simulink model "ROS_OAC_HOSM_Circular"  (R2018b)
settings: Solver=FixedStepAuto  StartTime=0.0  StopTime=inf  FixedStep=0.02  RelTol=1e-3
model workspace (MAT data in the model file):
  a = Simulink.Parameter
  a.DataType = 'auto'
  a.Dimensions = [0 0]
undefined symbols (not defined in the file): Angular, Linear, magnitude
libraries: simulink x3, robotlib x3
settings Model: Creator=Joru Fua  LastModifiedBy=Joru
settings OptimizationCC: EnhancedBackFolding=on  PassReuseOutputArgsAs=Individual arguments  MaxStackSize=64  OptimizeBlockOrder=speed  DifferentSizesBufferReuse=on  OptimizationCustomize=off
settings DebuggingCC: ParameterTunabilityLossMsg=error
settings HardwareCC: ProdBitPerPointer=32  ProdBitPerSizeT=32  ProdBitPerPtrDiffT=32  ProdLargestAtomicFloat=None  ProdIntDivRoundTo=Undefined  ProdEndianess=Unspecified  ProdWordSize=32  ProdHWDeviceType=Generic->Unspecified (assume 32-bit Generic)
settings SFSimCC: SimUseLocalCustomCode=off  MATLABDynamicMemAlloc=off
settings RTWCC: SystemTargetFile=ert.tlc  HardwareBoard=Robot Operating System (ROS)  TLCOptions="-aInlineSetEventsForThisBaseRateFcn=TLC_FALSE -aSuppressMultiTaskScheduler=TLC_FALSE  -aRateBasedStepFcn=0"  TemplateMakefile=ert_default_tmf  GenerateReport=on  RTWUseLocalCustomCode=off  Toolchain=Catkin  IncludeHyperlinkInReport=on  LaunchReport=on  TargetLang=C++  GenerateTraceInfo=on  GenerateTraceReport=on  GenerateTraceReportSl=on  GenerateTraceReportSf=on  GenerateTraceReportEml=on
settings CodeAppCC: ForceParamTrailComments=on  IgnoreCustomStorageClasses=off  OperatorAnnotations=on  SimulinkDataObjDesc=on  SFDataObjDesc=on  InsertBlockDesc=on
settings ERTTargetCC: SupportContinuousTime=on

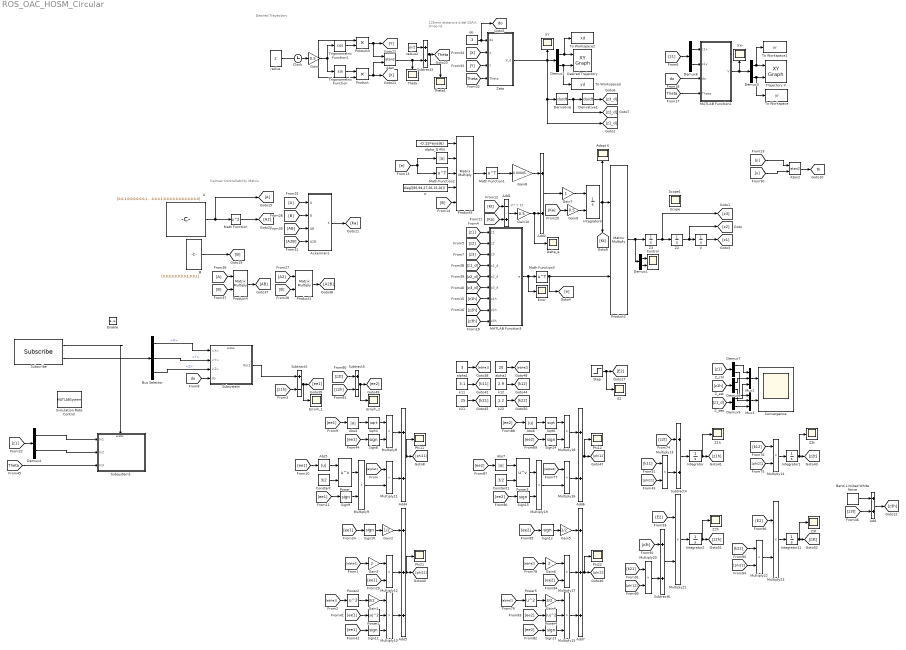
== system ROS_OAC_HOSM_Circular ==
  note: K* = Kt
  note: Kalman Controllability Matrix
  note: Desired Trayectory
  note: 125mm distancia d del SSAV;
      | 0<do<d
  Enable : EnablePort
  A : Constant  Value=[0,0,1,0,0,0;0,0,0,1,0,0;0,0,0,0,1,0;0,0,0,0,0,1;0,0,0,0,0,0;0,0,0,0,0,0]
  Abs{,4..7} (5 alike) : Abs
  Ackerman1 : MATLAB Function  TreatAsAtomicUnit=on
  Adapt K : Scope
  Add{,2,4,6} (4 alike) : Sum
  Add1 : Sum  Inputs=-+
  Add5 : Sum  Inputs=+++
  Add7 : Sum  Inputs=+++
  Atan : Trigonometry  Operator=atan2
  Atan2 : Trigonometry  Operator=atan2
  B : Constant  Value=[0,0;0,0;0,0;0,0;1,0;0,1]  VectorParams1D=off
  Band-Limited White Noise : simulink/Sources/Band-Limited White Noise  Cov=[0.00001]  Ts=0.02  seed=[23341]
  Bus Selector : BusSelector  OutputSignals=Pose.Pose.Position.X,Pose.Pose.Position.Y,Twist.Twist.Angular.Z
  Clock : Clock
  Constant : Constant  Value=3/2
  Constant1 : Constant  Value=3/2
  Control : Scope  NumInputPorts=2
  Convergence : Scope  NumInputPorts=2
  Delta_e : Scope
  Demux{1..4,6..9} (8 alike) : Demux  Outputs=2
  Derivative : Derivative
  Derivative1 : Derivative
  Desired Trajectory : simulink/Sinks/XY Graph  xmin=-5  xmax=5  ymin=-5  ymax=5  st=.1
  E2 : Scope
  Error : Scope
  Errorh_1 : Scope
  Errorh_2 : Scope
  Gain : Gain  Gain=0.5
  Gain1 : Gain  Gain=3/2
  Gain10 : Gain  Gain=0.5
  Gain2 : Gain  Gain=1/2
  Gain3 : Gain  Gain=2
  Gain4 : Gain  Gain=3/2
  Gain5 : Gain  Gain=1/2
  Gain6 : Gain  Gain=2
  Gain7 : Gain
  Gain8 : Gain  Gain=0.00005
  Gain9 : Gain  Gain=0.5
  Integrator{,1..2,11} (4 alike) : Integrator  InitialCondition=[0;0]
  Integrator3 : Integrator  InitialConditionSource=external  InitialCondition=[0.3148,1.3520,2.7441,3.3146,2.4323,0.9017;0.0296,0.1557,0.4075,0.7024,0.9017,1.0442];
  MATLAB Function2 : MATLAB Function  TreatAsAtomicUnit=on
  MATLAB Function3 : MATLAB Function  TreatAsAtomicUnit=on
  Math Function : Math  Operator=square  SaturateOnIntegerOverflow=on
  Math Function1 : Math  Operator=transpose  SaturateOnIntegerOverflow=on
  Math Function2 : Math  Operator=transpose  SaturateOnIntegerOverflow=on
  Math Function3 : Math  Operator=transpose  SaturateOnIntegerOverflow=on
  Multiply10 : Product  Inputs=3
  Multiply{8..9,11..14,16..23} (14 alike) : Product
  Multiply15 : Product  Inputs=3
  Mux2 : Mux  Inputs=3
  Mux3 : Mux  Inputs=3
  P : Constant  Value=diag([85,94,27,26,15,26])
  Phi{11..12,21..22} (4 alike) : Scope
  Power : Math  Operator=pow  SaturateOnIntegerOverflow=on
  Power1 : Math  Operator=magnitude^2  SaturateOnIntegerOverflow=on
  Power2 : Math  Operator=square  SaturateOnIntegerOverflow=on
  Power3 : Math  Operator=pow  SaturateOnIntegerOverflow=on
  Power4 : Math  Operator=magnitude^2  SaturateOnIntegerOverflow=on
  Power5 : Math  Operator=square  SaturateOnIntegerOverflow=on
  Product : Product
  Product1 : Product  Multiplication=Matrix(*)
  Product2 : Product  Multiplication=Matrix(*)
  Product3 : Product
  Product4 : Product  Multiplication=Matrix(*)
  Product5 : Product  Inputs=5  Multiplication=Matrix(*)
  Sign{8..15} (8 alike) : Signum
  Simulation Rate Control : MATLABSystem  System=ExampleHelperSimulationRateControl  SampleTime=0.02
      mask Type: ExampleHelperSimulationRateControl
      mask Display: disp('Rate Control');
  Sqrt4 : Sqrt  SaturateOnIntegerOverflow=on
  Sqrt6 : Sqrt  SaturateOnIntegerOverflow=on
  Step : Step  Time=0.000000001  SampleTime=0.02
  Subscribe : robotlib/Subscribe  topicSource=Specify your own  topic=/odom  messageType=nav_msgs/Odometry  sampleTime=-1  messageQueueLength=1
      settings: SourceProductBaseCode=RO
  Subsystem : Subsystem
  Subsystem1 : Subsystem
  Subtract2 : Sum  Inputs=+-
  Subtract3 : Sum
  Subtract4 : Sum
  Subtract5 : Sum  Inputs=+-
  Subtract6 : Sum
  Theta : Scope
  Theta1 : Scope
  To Workspace : ToWorkspace  VariableName=yr  SampleTime=-1
      settings: Save2DSignal=2-D array (concatenate along first dimension)
  To Workspace1 : ToWorkspace  VariableName=xr  SampleTime=-1
      settings: Save2DSignal=2-D array (concatenate along first dimension)
  To Workspace2 : ToWorkspace  VariableName=xd  SampleTime=-1
      settings: Save2DSignal=2-D array (concatenate along first dimension)
  To Workspace3 : ToWorkspace  VariableName=yd  SampleTime=-1
      settings: Save2DSignal=2-D array (concatenate along first dimension)
  Trajectory V : simulink/Sinks/XY Graph  xmin=-5  xmax=5  ymin=-5  ymax=5  st=.1
  Trigonometric Function : Trigonometry
  Trigonometric Function1 : Trigonometry  Operator=cos
  V : Integrator  InitialCondition=[0;0]
  XY : Scope
  XYr : Scope
  Z1h : Scope
  Z2 : Integrator  InitialCondition=[0;0]
  Z2h : Scope
  Z2t : Scope
  Z3 : Integrator  InitialCondition=[0;0]
  Z3t : Scope
  Zeta : MATLAB Function  TreatAsAtomicUnit=on
  alpha1 : Constant  Value=3
  alpha2 : Constant  Value=20
  alpha_Q : Constant  Value=-0.15*eye(6)
  do : Constant  Value=.3
  k11 : Constant  Value=3.1
  k12 : Constant  Value=2.9
  k21 : Constant  Value=.25
  k22 : Constant  Value=1.2
  radius : Constant  Value=2
  radius2 : Constant  Value=pi/2
  Scope : Scope
  Scope1 : Scope
  tag scope: Theta=global, do=global, th=global
  wires:
  Z3/1 -> [z3], Z2/1
  V/1 -> [z1]
  Derivative1/1 -> [z3_d]
  Derivative/1 -> [z2_d], Derivative1/1
  Product2/1 -> Demux1/1, Z3/1
  Zeta/1(V_d) -> Demux2/1, XY/1, Derivative/1, [z1_d]
  [Theta] -> MATLAB Function2/4(Theta)
  [do] -> MATLAB Function2/3(do)
  Demux6/1 -> MATLAB Function2/1(z1x)
  Demux6/2 -> MATLAB Function2/2(z1y)
  Atan/1 -> Subtract3/2, Theta/1
  radius2/1 -> Subtract3/1
  do/1 -> [do], Zeta/1(do)
  Product/1 -> [X], Atan/2
  Clock/1 -> Gain/1
  [Theta] -> Zeta/4(Theta)
  [X] -> Zeta/2(X)
  [Y] -> Zeta/3(Y)
  Gain/1 -> Trigonometric Function/1, Trigonometric Function1/1
  Trigonometric Function/1 -> Product/1
  radius/1 -> Product/2, Product3/1
  Product3/1 -> Atan/1, [Y]
  Trigonometric Function1/1 -> Product3/2
  [A] -> Ackerman1/1(A)
  B/1 -> [B]
  [AB] -> Ackerman1/3(AB)
  [B] -> Product1/2
  [B] -> Ackerman1/2(B)
  Math Function/1 -> [A2]
  [A2B] -> Ackerman1/4(A2B)
  A/1 -> [A], Math Function/1
  [A2] -> Product1/1
  Product1/1 -> [A2B]
  Product4/1 -> [AB]
  [B] -> Product4/2
  [A] -> Product4/1
  [z3] -> MATLAB Function3/3(z3)
  [z2] -> MATLAB Function3/2(z2)
  [z1] -> MATLAB Function3/1(z1)
  [z1_d] -> MATLAB Function3/4(z1_d)
  [z2_d] -> MATLAB Function3/5(z2_d)
  [z3_d] -> MATLAB Function3/6(z3_d)
  MATLAB Function2/1(V) -> Demux3/1, XYr/1
  Demux3/1 -> To Workspace1/1, Trajectory V/1
  Demux3/2 -> To Workspace/1, Trajectory V/2
  Demux2/1 -> Desired Trajectory/1, To Workspace2/1
  Demux2/2 -> To Workspace3/1, Desired Trajectory/2
  Abs4/1 -> Sqrt4/1
  Constant/1 -> Power/2
  Sqrt4/1 -> Multiply8/1
  Sign8/1 -> Multiply8/2
  Power/1 -> Multiply9/1
  Sign9/1 -> Multiply9/2
  Multiply8/1 -> Add4/1
  Add4/1 -> Phi11/1, [phi11]
  Sign10/1 -> Gain2/1
  Gain2/1 -> Add5/1
  Multiply10/1 -> Add5/3
  Sign11/1 -> Multiply10/3
  alpha1/1 -> [alpha1]
  Multiply9/1 -> Multiply11/2
  [alpha1] -> Multiply11/1
  Multiply11/1 -> Add4/2
  [alpha1] -> Gain3/1
  Gain3/1 -> Multiply12/1
  Multiply12/1 -> Add5/2
  Gain1/1 -> Multiply10/1
  Power2/1 -> Gain1/1
  [alpha1] -> Power2/1
  Power1/1 -> Multiply10/2
  Subtract2/1 -> Errorh_1/1, [ee1]
  [ee1] -> Abs4/1
  [ee1] -> Abs5/1
  [ee1] -> Sign9/1
  [ee1] -> Sign10/1
  [ee1] -> Multiply12/2
  [ee1] -> Power1/1
  [ee1] -> Sign11/1
  [ee1] -> Sign8/1
  k11/1 -> [k11]
  Subtract4/1 -> Integrator/1
  Integrator/1 -> Z1h/1, [z1h]
  Multiply14/1 -> Integrator1/1
  Integrator1/1 -> Z2t/1, [z2t]
  k12/1 -> [k12]
  k21/1 -> [k21]
  [ee2] -> Sign14/1
  Add7/1 -> Phi22/1, [phi22]
  [ee2] -> Sign13/1
  [ee2] -> Power4/1
  [ee2] -> Multiply17/2
  [ee2] -> Sign12/1
  [ee2] -> Sign15/1
  [ee2] -> Abs7/1
  [ee2] -> Abs6/1
  Power4/1 -> Multiply15/2
  [alpha2] -> Power5/1
  Power5/1 -> Gain4/1
  Gain4/1 -> Multiply15/1
  Multiply17/1 -> Add7/2
  Gain6/1 -> Multiply17/1
  [alpha2] -> Gain6/1
  Multiply16/1 -> Add6/2
  [alpha2] -> Multiply16/1
  Multiply19/1 -> Multiply16/2
  Sign13/1 -> Multiply15/3
  Multiply15/1 -> Add7/3
  Gain5/1 -> Add7/1
  Sign12/1 -> Gain5/1
  Add6/1 -> Phi12/1, [phi12]
  Multiply18/1 -> Add6/1
  Sign15/1 -> Multiply19/2
  Power3/1 -> Multiply19/1
  Sign14/1 -> Multiply18/2
  Sqrt6/1 -> Multiply18/1
  Constant1/1 -> Power3/2
  Abs6/1 -> Sqrt6/1
  alpha2/1 -> [alpha2]
  Subtract5/1 -> Errorh_2/1, [ee2]
  k22/1 -> [k22]
  [phi11] -> Multiply13/2
  [k11] -> Multiply13/1
  Multiply13/1 -> Subtract4/2
  [z2t] -> Subtract4/1
  [k12] -> Multiply14/1
  [phi21] -> Multiply14/2
  [z3t] -> Subtract6/1
  Multiply20/1 -> Subtract6/2
  [k21] -> Multiply20/1
  [phi12] -> Multiply20/2
  Integrator2/1 -> Z2h/1, [z2h]
  Subtract6/1 -> Multiply21/2
  [E2] -> Multiply21/1
  Multiply21/1 -> Integrator2/1
  [phi22] -> Multiply22/2
  [k22] -> Multiply22/1
  Multiply22/1 -> Multiply23/2
  [E2] -> Multiply23/1
  Integrator11/1 -> [z3t], Z3t/1
  Multiply23/1 -> Integrator11/1
  [z1h] -> MATLAB Function3/7(z1h)
  [z2h] -> MATLAB Function3/8(z2h)
  [z3h] -> MATLAB Function3/9(z3h)
  Step/1 -> E2/1, [E2]
  Add5/1 -> Phi21/1, [phi21]
  [z1h] -> Subtract2/2
  [z2t] -> Subtract5/1
  [z2h] -> Subtract5/2
  Abs5/1 -> Power/1
  Abs7/1 -> Power3/1
  Z2/1 -> [z2], V/1
  Band-Limited White Noise/1 -> Add/1
  Add/1 -> [z3h]
  [z3t] -> Add/2
  Mux2/1 -> Convergence/1
  Mux3/1 -> Convergence/2
  [z1] -> Demux7/1
  [z1h] -> Demux8/1
  [z1_d] -> Demux9/1
  Demux7/1 -> Mux2/1
  Demux8/1 -> Mux2/2
  Demux9/1 -> Mux2/3
  Demux7/2 -> Mux3/1
  Demux9/2 -> Mux3/3
  Demux8/2 -> Mux3/2
  Demux1/1 -> Control/1
  Demux1/2 -> Control/2
  [z1] -> Demux6/1
  Add2/1 -> Gain7/1
  alpha_Q/1 -> Product5/1
  P/1 -> Product5/4
  Integrator3/1 -> Product2/1, Adapt K/1, [Kt]
  [B] -> Product5/5
  Add1/1 -> Gain10/1
  MATLAB Function3/1(e) -> Error/1, Math Function3/1
  Ackerman1/1(K) -> [Ka]
  Product5/1 -> Math Function1/1
  Math Function3/1 -> Product2/2, [e]
  Math Function2/1 -> Product5/3
  [Kt] -> Add1/1
  Math Function1/1 -> Gain8/1
  [Ka] -> Gain9/1
  Gain7/1 -> Integrator3/1
  [Ka] -> Add1/2
  Gain9/1 -> Integrator3/2
  Gain8/1 -> Add2/1
  Gain10/1 -> Delta_e/1, Add2/2
  [e] -> Abs/1, Math Function2/1
  Abs/1 -> Product5/2
  [y] -> Atan2/1
  [x] -> Atan2/2
  Atan2/1 -> [th]
  Subtract3/1 -> Theta1/1, [Theta]
  [z1] -> Demux4/1
  Subscribe/1 -> Subsystem1/Enable
  Subscribe/2 -> Bus Selector/1
  Bus Selector/1 -> Subsystem/1(<X>)  "<X>"
  Bus Selector/2 -> Subsystem/2(<Y>)  "<Y>"
  Bus Selector/3 -> Subsystem/3(<Z>)  "<Z>"
  Subsystem/1(Out1) -> Subtract2/1
  Demux4/1 -> Subsystem1/1(In1)
  Demux4/2 -> Subsystem1/2(In2)
  [Theta] -> Subsystem1/3(In3)
  [do] -> Subsystem/4(do)

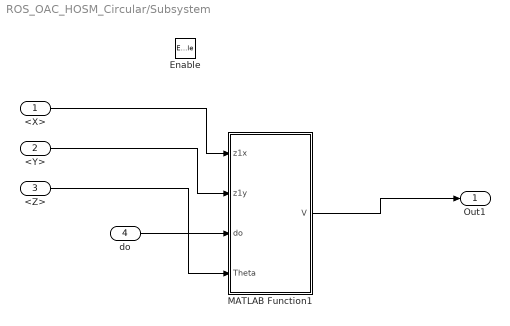
== system ROS_OAC_HOSM_Circular/Subsystem ==
  <X> : Inport
  <Y> : Inport  Port=2
  <Z> : Inport  Port=3
  do : Inport  Port=4
  Enable : EnablePort
  MATLAB Function1 : MATLAB Function  TreatAsAtomicUnit=on
  Out1 : Outport
  wires:
  do/1 -> MATLAB Function1/3(do)
  MATLAB Function1/1(V) -> Out1/1
  <Y>/1 -> MATLAB Function1/2(z1y)
  <Z>/1 -> MATLAB Function1/4(Theta)
  <X>/1 -> MATLAB Function1/1(z1x)

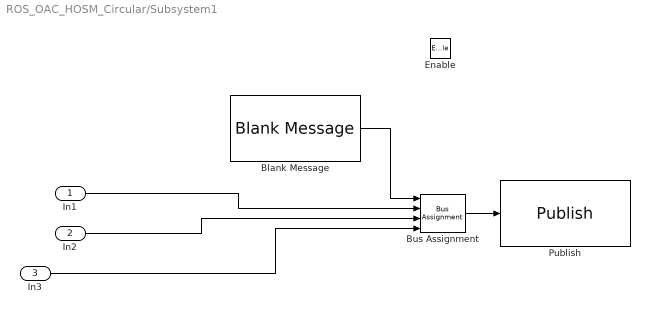
== system ROS_OAC_HOSM_Circular/Subsystem1 ==
  In1 : Inport
  In2 : Inport  Port=2
  In3 : Inport  Port=3
  Enable : EnablePort
  Blank Message : robotlib/Blank Message  messageClass=Message  entityType=geometry_msgs/Twist  messageType=geometry_msgs/Twist  SampleTime=inf
      settings: SourceProductBaseCode=RO
  Bus Assignment : BusAssignment  AssignedSignals=Linear.X,Linear.Y,Angular.Z
  Publish : robotlib/Publish  topicSource=Specify your own  topic=/cmd_vel  messageType=geometry_msgs/Twist  messageQueueLength=1
      link override SinkBlock: ROSTopic=/cmd_vel  ROSMessageType=geometry_msgs/Twist  SLBusName=SL_Bus_OAC_HOSM_Circular_geometry_msgs_Twist  ModelName=OAC_HOSM_Circular  BlockId=Pub_OAC_HOSM_Circular_1235
      settings: SourceProductBaseCode=RO
  wires:
  In2/1 -> Bus Assignment/3
  Blank Message/1 -> Bus Assignment/1
  Bus Assignment/1 -> Publish/1
  In1/1 -> Bus Assignment/2
  In3/1 -> Bus Assignment/4

== matlab function ROS_OAC_HOSM_Circular/Subsystem/MATLAB Function1 ==
  data: z1x input; z1y input; do input; V output; Theta input
function V = fcn(z1x,z1y,do,Theta)

x = z1x; %+ do*cos(Theta);
y = z1y; %+ do*sin(Theta);

V = [x;
     y];

== matlab function ROS_OAC_HOSM_Circular/Ackerman1 ==
  data: A input; K output; B input; AB input; A2B input
function K = fcn(A,B,AB,A2B)
% C = [B,AB,A2B];
% JA=poly(A);
% a1=JA(2);a2=JA(3);a3=JA(4);
% W= [a2,a1,1;a1,1,0;1,0,0];
% T=C*W;
% J=[-2+j*4, -2-j*4, -10];
% JJ=poly(J);
% aa1=JJ(2); aa2=JJ(3); aa3=JJ(4);
% k=[aa3-a3,aa2-a2,aa1-a1];

%Ackerman
%malK = [-200,-60,-14];

%LQR
%malK = [-1 -2.4142 -2.4142];
%[K,S,e] = lqr(A,B,eye(6),eye(2))
%-1*place(A,B,[-15 -10 -12 -14 -17 -19])

%Ko=-1*lqr(A,B,1.9*diag([5 6 7 3 4 5]),0.9*diag([4 7]))
K=[-1.62446572413483,0,-3.70380724394541,0,-3.08524319932836,0;0,-1.34518541826910,0,-2.85111979498417,0,-2.68517710736273]

== matlab function ROS_OAC_HOSM_Circular/Zeta ==
  data: do input; X input; V_d output; Y input; Theta input
function V_d = fcn(do,X,Y,Theta)

V_d = [X + do*cos(Theta);
       Y + do*sin(Theta)];

== matlab function ROS_OAC_HOSM_Circular/MATLAB Function3 ==
  data: z1 input; e output; z2 input; z3 input; z1_d input; z2_d input; z3_d input; z1h input; z2h input; z3h input
function e = fcn(z1,z2,z3,z1_d,z2_d,z3_d,z1h,z2h,z3h)

w = [z1;z2;z3];

w_d = [z1_d;z2_d;z3_d];

wh = [z1h;z2h;z3h];

%e = w' - w_d';

e = wh' - w_d';

== matlab function ROS_OAC_HOSM_Circular/MATLAB Function2 ==
  data: z1x input; z1y input; do input; V output; Theta input
function V = fcn(z1x,z1y,do,Theta)

x = z1x; %+ do*cos(Theta);
y = z1y; %+ do*sin(Theta);

V = [x;
     y];
